simulink library "csc_rsp_radar_sensor_prep_lib"  (R2015b)
settings: Solver=ode45  SolverMode=SingleTasking  StartTime=0.0  StopTime=10.0  RelTol=1e-3
values from neighbouring files (symbols this model uses):
  rsp_ldr1_lander_dcm = rot_angles_to_dcm( [rsp_ldr1_lander_rotz rsp_ldr1_lander_roty rsp_ldr1_lander_rotx] )    [csc_rsp_radar_sensor_prep.m]
  snp_rdr_index = [ 1 2 ]    [csc_snp_sensor_prep_init.m]
  snp_rdr_zero_index = [ 0 0 ]    [csc_snp_sensor_prep_init.m]
undefined symbols (not defined in the file or in its folder): accel, central_body_flattening, central_body_radius, central_body_rotation_rate, ini_topocentric_latitude, kfl_target_site_planet_fixed, kfl_topo_z_to_alt, kfl_use_range_meas, q, x
libraries: util_common_lib x15, simulink x12, util_frame_rotation_lib x7, simulink_extras x6, util_quat_lib x5, util_fsw_frame_rotation_lib x5, util_geodesy_lib x4, util_info_lib x3, csu_und_unduplicate_lib x3, csc_rsp_radar_sensor_prep_lib x2
settings Model: ExtModeAutoUpdateStatusClock=off  Creator=Administrator  LastModifiedBy=Mark Agbayani
settings DataIOCC: SaveFormat=Array  SignalLoggingSaveFormat=ModelDataLogs
settings OptimizationCC: BlockReduction=off  BooleanDataType=off  ExpressionDepthLimit=2147483647
settings DebuggingCC: SaveWithParameterizedLinksMsg=none  UnderspecifiedInitializationDetection=Classic  MergeDetectMultiDrivingBlocksExec=none  SignalResolutionControl=TryResolveAllWithWarning  FcnCallInpInsideContextMsg=EnableAllAsWarning  StateNameClashWarn=warning  StrictBusMsg=Warning
settings HardwareCC: ProdBitPerPointer=32  ProdLargestAtomicFloat=None  ProdIntDivRoundTo=Undefined  ProdEndianess=Unspecified  ProdWordSize=32  ProdHWDeviceType=32-bit Generic  TargetUnknown=on
settings GRTTargetCC: GeneratePreprocessorConditionals=Disable all  CombineOutputUpdateFcns=off  GRTInterface=on
settings ConfigComp: CovModelRefEnable=Off  CovSFcnEnable=off

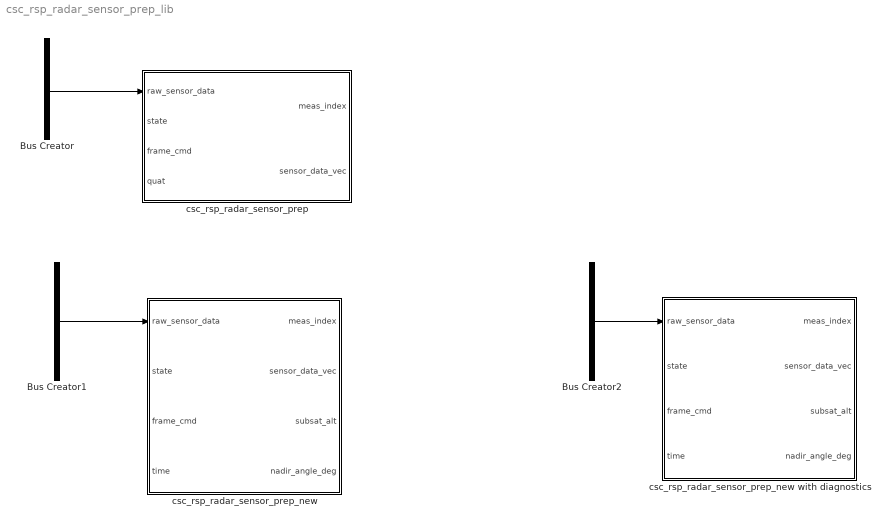
== system csc_rsp_radar_sensor_prep_lib ==
  Bus Creator : BusCreator  Inputs=4
  Bus Creator1 : BusCreator  Inputs=5
  Bus Creator2 : BusCreator  Inputs=5
  csc_rsp_radar_sensor_prep : Subsystem
  csc_rsp_radar_sensor_prep_new : Subsystem
  csc_rsp_radar_sensor_prep_new with diagnostics : Subsystem
  wires:
  ? -> Bus Creator/2  "accel"
  ? -> Bus Creator/3  "rate"
  ? -> Bus Creator/1  "x"
  ? -> Bus Creator/4  "q"
  Bus Creator/1 -> csc_rsp_radar_sensor_prep/1(raw_sensor_data)
  ? -> Bus Creator1/2  "accel"
  ? -> Bus Creator1/3  "rate"
  ? -> Bus Creator1/1  "x"
  ? -> Bus Creator1/4  "q"
  Bus Creator1/1 -> csc_rsp_radar_sensor_prep_new/1(raw_sensor_data)
  ? -> Bus Creator1/5  "altitude"
  ? -> Bus Creator2/2  "accel"
  ? -> Bus Creator2/3  "rate"
  ? -> Bus Creator2/1  "x"
  ? -> Bus Creator2/4  "q"
  Bus Creator2/1 -> csc_rsp_radar_sensor_prep_new with diagnostics/1(raw_sensor_data)
  ? -> Bus Creator2/5  "altitude"

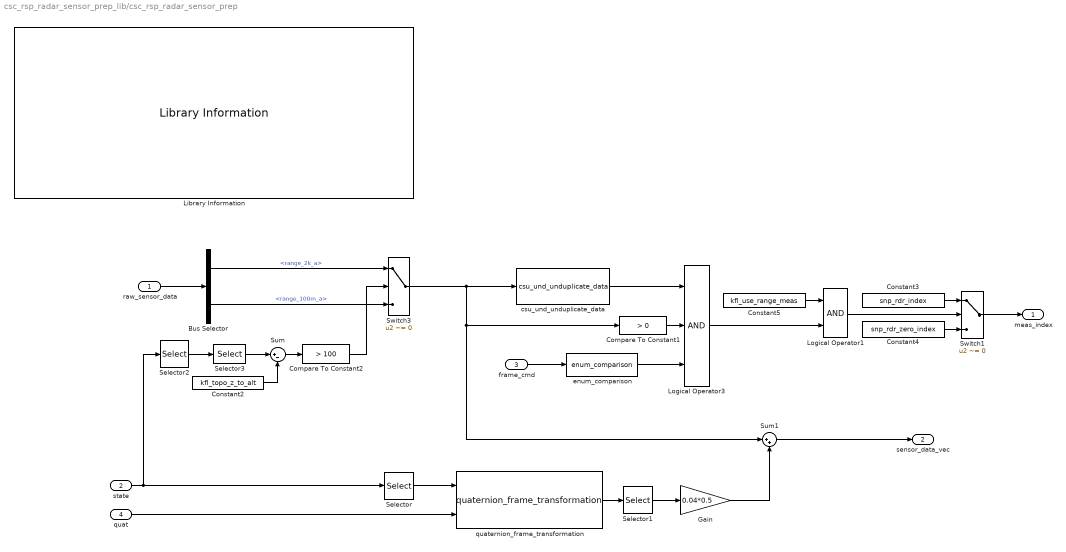
== system csc_rsp_radar_sensor_prep_lib/csc_rsp_radar_sensor_prep ==
  raw_sensor_data : Inport
  state : Inport  Port=2
  frame_cmd : Inport  Port=3
  quat : Inport  Port=4
  Bus Selector : BusSelector  OutputSignals=range_2k_a,range_100m_a
  Compare To Constant1 : simulink/Logic and Bit Operations/Compare To Constant  relop=>  const=0  OutDataTypeStr=uint8
  Compare To Constant2 : simulink/Logic and Bit Operations/Compare To Constant  relop=>  const=100  OutDataTypeStr=uint8
  Constant2 : Constant  Value=kfl_topo_z_to_alt
  Constant3 : Constant  Value=snp_rdr_index
  Constant4 : Constant  Value=snp_rdr_zero_index
  Constant5 : Constant  Value=kfl_use_range_meas
  Gain : Gain  Gain=0.04*0.5
  Library Information : util_info_lib/Library Information  owner='NONE'
  Logical Operator1 : Logic  AllPortsSameDT=off  OutDataTypeStr=boolean
  Logical Operator3 : Logic  Inputs=3  AllPortsSameDT=off  OutDataTypeStr=boolean
  Selector : Selector  InputPortWidth=kfl_n_state  IndexOptions=Index vector (dialog)  Indices=kfl_vel_index  OutputSizes=1
  Selector1 : Selector  InputPortWidth=3  IndexOptions=Index vector (dialog)  Indices=3  OutputSizes=1
  Selector2 : Selector  InputPortWidth=kfl_n_state  IndexOptions=Index vector (dialog)  Indices=kfl_pos_index  OutputSizes=1
  Selector3 : Selector  InputPortWidth=3  IndexOptions=Index vector (dialog)  Indices=[3]  OutputSizes=1
  Sum : Sum  Inputs=|+-
  Sum1 : Sum  Inputs=|++
  Switch1 : Switch  Criteria=u2 ~= 0
  Switch3 : Switch  Criteria=u2 ~= 0
  csu_und_unduplicate_data : csu_und_unduplicate_lib/csu_und_unduplicate_data  initial_compare=0
  enum_comparison : util_common_lib/enum_comparison  comparison_type===
  quaternion_frame_transformation : util_quat_lib/quaternion_frame_transformation  SystemSampleTime=-1
  meas_index : Outport
  sensor_data_vec : Outport  Port=2
  wires:
  csu_und_unduplicate_data/1 -> Logical Operator3/1
  Constant5/1 -> Logical Operator1/1
  Logical Operator1/1 -> Switch1/2
  Logical Operator3/1 -> Logical Operator1/2
  Constant4/1 -> Switch1/3
  Constant3/1 -> Switch1/1
  Switch3/1 -> csu_und_unduplicate_data/1, Compare To Constant1/1, Sum1/1
  Bus Selector/2 -> Switch3/3  "<range_100m_a>"
  Bus Selector/1 -> Switch3/1  "<range_2k_a>"
  Compare To Constant2/1 -> Switch3/2
  Sum/1 -> Compare To Constant2/1
  Selector2/1 -> Selector3/1
  Constant2/1 -> Sum/2
  Selector3/1 -> Sum/1
  Sum1/1 -> sensor_data_vec/1
  Gain/1 -> Sum1/2
  Selector1/1 -> Gain/1
  quaternion_frame_transformation/1 -> Selector1/1
  quat/1 -> quaternion_frame_transformation/2
  Selector/1 -> quaternion_frame_transformation/1
  state/1 -> Selector/1, Selector2/1
  frame_cmd/1 -> enum_comparison/1
  Compare To Constant1/1 -> Logical Operator3/2
  raw_sensor_data/1 -> Bus Selector/1
  Switch1/1 -> meas_index/1
  enum_comparison/1 -> Logical Operator3/3

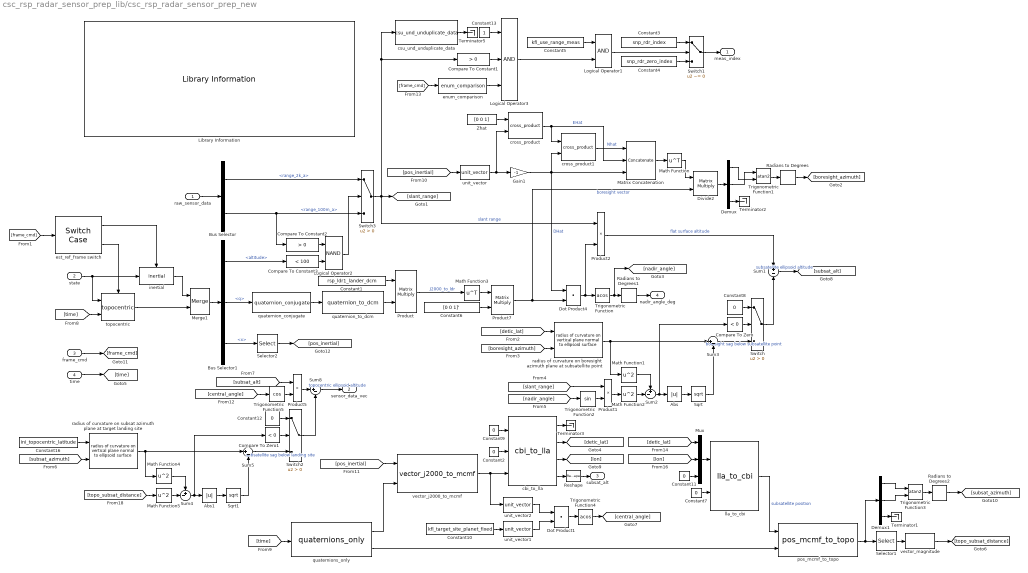
== system csc_rsp_radar_sensor_prep_lib/csc_rsp_radar_sensor_prep_new ==
  raw_sensor_data : Inport
  state : Inport  Port=2
  frame_cmd : Inport  Port=3
  time : Inport  Port=4
  Abs : Abs
  Abs1 : Abs
  Bus Selector : BusSelector  OutputSignals=range_2k_a,range_100m_a
  Bus Selector1 : BusSelector  OutputSignals=altitude,q,x
  Compare To Constant1 : simulink/Logic and Bit Operations/Compare To Constant  relop=>  const=0  OutDataTypeStr=uint8
  Compare To Constant2 : simulink/Logic and Bit Operations/Compare To Constant  relop=>  const=0  OutDataTypeStr=uint8
  Compare To Constant3 : simulink/Logic and Bit Operations/Compare To Constant  relop=<  const=100  OutDataTypeStr=uint8
  Compare To Zero : simulink/Logic and Bit Operations/Compare To Zero  relop=<  OutDataTypeStr=boolean
  Compare To Zero1 : simulink/Logic and Bit Operations/Compare To Zero  relop=<  OutDataTypeStr=boolean
  Constant1 : Constant  Value=rsp_ldr1_lander_dcm
  Constant10 : Constant  Value=kfl_target_site_planet_fixed
  Constant{2,7..9,11..12} (6 alike) : Constant  Value=0
  Constant13 : Constant  OutDataTypeStr=boolean
  Constant16 : Constant  Value=ini_topocentric_latitude
  Constant3 : Constant  Value=snp_rdr_index
  Constant4 : Constant  Value=snp_rdr_zero_index
  Constant5 : Constant  Value=kfl_use_range_meas
  Constant6 : Constant  Value=[0 0 1]'  VectorParams1D=off
  Demux : Demux  Outputs=3
  Demux1 : Demux  Outputs=3
  Divide2 : Product  Inputs=**  Multiplication=Matrix(*)
  Dot Product1 : DotProduct  InputSameDT=on  OutDataTypeStr=Inherit: Inherit via internal rule
  Dot Product4 : DotProduct  InputSameDT=on  OutDataTypeStr=Inherit: Inherit via internal rule
  Gain1 : Gain  Gain=-1
  Library Information : util_info_lib/Library Information  owner='NONE'
  Logical Operator1 : Logic  AllPortsSameDT=off  OutDataTypeStr=boolean
  Logical Operator2 : Logic  Operator=NAND  AllPortsSameDT=off  OutDataTypeStr=boolean
  Logical Operator3 : Logic  Inputs=3  AllPortsSameDT=off  OutDataTypeStr=boolean
  Math Function : Math  Operator=transpose  SaturateOnIntegerOverflow=on
  Math Function{1..2,4..5} (4 alike) : Math  Operator=square  SaturateOnIntegerOverflow=on
  Math Function3 : Math  Operator=transpose  SaturateOnIntegerOverflow=on
  Matrix Concatenation : Concatenate  NumInputs=3  Mode=Multidimensional array  ConcatenateDimension=2
  Merge1 : Merge  InitialOutput=0
  Mux : Mux  Inputs=3
  Product : Product  Multiplication=Matrix(*)  RndMeth=Zero
  Product1 : Product  Inputs=**  RndMeth=Zero
  Product2 : Product  Inputs=**  RndMeth=Zero
  Product5 : Product  Inputs=**  RndMeth=Zero
  Product7 : Product  Multiplication=Matrix(*)  RndMeth=Zero
  Radians to Degrees : simulink_extras/Transformations/Radians to Degrees
  Radians to Degrees1 : simulink_extras/Transformations/Radians to Degrees
  Radians to Degrees2 : simulink_extras/Transformations/Radians to Degrees
  Reshape : Reshape
  Selector1 : Selector  InputPortWidth=3  IndexOptions=Index vector (dialog)  Indices=[1 2]  OutputSizes=1
  Selector2 : Selector  InputPortWidth=kfl_n_state  IndexOptions=Index vector (dialog)  Indices=kfl_pos_index  OutputSizes=1
  Sqrt : Sqrt  SaturateOnIntegerOverflow=on
  Sqrt1 : Sqrt  SaturateOnIntegerOverflow=on
  Sum1 : Sum  Inputs=+|-
  Sum2 : Sum  Inputs=+-|  AccumDataTypeStr=double
  Sum3 : Sum  Inputs=|+-
  Sum4 : Sum  Inputs=+-|  AccumDataTypeStr=double
  Sum5 : Sum  Inputs=|+-
  Sum8 : Sum  Inputs=|+-
  Switch : Switch  Criteria=u2 > Threshold
  Switch1 : Switch  Criteria=u2 ~= 0
  Switch2 : Switch  Criteria=u2 > Threshold
  Switch3 : Switch  Criteria=u2 > Threshold
  Terminator{1..3,5} (4 alike) : Terminator
  Trigonometric Function : Trigonometry  Operator=acos
  Trigonometric Function1 : Trigonometry  Operator=atan2
  Trigonometric Function2 : Trigonometry
  Trigonometric Function3 : Trigonometry  Operator=atan2
  Trigonometric Function4 : Trigonometry  Operator=acos
  Trigonometric Function5 : Trigonometry  Operator=cos
  Zhat : Constant  Value=[0 0 1]
  cbi_to_lla : util_frame_rotation_lib/cbi_to_lla  a=central_body_radius  b=central_body_radius*(1-central_body_flattening)  omega=central_body_rotation_rate(3)
  cross_product : util_common_lib/cross_product  SystemSampleTime=-1
  cross_product1 : util_common_lib/cross_product  SystemSampleTime=-1
  csu_und_unduplicate_data : csu_und_unduplicate_lib/csu_und_unduplicate_data  initial_compare=0
  enum_comparison : util_common_lib/enum_comparison  comparison_type===
  est_ref_frame switch : SwitchCase  CaseConditions={uint8(enum_reference_frame.inertial),uint8(enum_reference_frame.topocentric)}  ShowDefaultCase=off
  inertial : csc_rsp_radar_sensor_prep_lib/csc_rsp_radar_sensor_prep_new with diagnostics/inertial
  lla_to_cbi : util_frame_rotation_lib/lla_to_cbi  a=central_body_radius  b=central_body_radius*(1-central_body_flattening)
  pos_mcmf_to_topo : util_fsw_frame_rotation_lib/pos_mcmf_to_topo  SystemSampleTime=-1
  quaternion_conjugate : util_quat_lib/quaternion_conjugate  SystemSampleTime=-1
  quaternion_to_dcm : util_quat_lib/quaternion_to_dcm  SystemSampleTime=-1
  quaternions_only : util_frame_rotation_lib/quaternions_only  SystemSampleTime=-1
  radius of curvature on boresight azimuth plane at subsatellite point : util_geodesy_lib/radius of curvature on vertical plane normal to ellipsoid surface  a=central_body_radius  b=central_body_radius*(1-central_body_flattening)
  radius of curvature on subsat azimuth plane at target landing site : util_geodesy_lib/radius of curvature on vertical plane normal to ellipsoid surface  a=central_body_radius  b=central_body_radius*(1-central_body_flattening)
  topocentric : csc_rsp_radar_sensor_prep_lib/csc_rsp_radar_sensor_prep_new with diagnostics/topocentric
  unit_vector : util_common_lib/unit_vector  SystemSampleTime=-1
  unit_vector1 : util_common_lib/unit_vector  SystemSampleTime=-1
  unit_vector2 : util_common_lib/unit_vector  SystemSampleTime=-1
  vector_j2000_to_mcmf : util_fsw_frame_rotation_lib/vector_j2000_to_mcmf  SystemSampleTime=-1
  vector_magnitude : util_common_lib/vector_magnitude  SystemSampleTime=-1
  meas_index : Outport
  sensor_data_vec : Outport  Port=2
  subsat_alt : Outport  Port=3
  nadir_angle_deg : Outport  Port=4
  wires:
  Reshape/1 -> subsat_alt/1
  Switch3/1 -> [slant_range], csu_und_unduplicate_data/1, Compare To Constant1/1, Product2/1  "slant range"
  unit_vector2/1 -> Dot Product1/1
  [pos_inertial] -> unit_vector/1
  Selector2/1 -> [pos_inertial]
  [pos_inertial] -> vector_j2000_to_mcmf/1
  unit_vector1/1 -> Dot Product1/2
  Constant11/1 -> Mux/3
  [detic_lat] -> Mux/1
  [lon] -> Mux/2
  cbi_to_lla/2 -> [detic_lat]
  cbi_to_lla/3 -> [lon]
  cbi_to_lla/1 -> Terminator3/1
  Constant9/1 -> cbi_to_lla/1
  Constant2/1 -> cbi_to_lla/2
  vector_j2000_to_mcmf/1 -> cbi_to_lla/3, unit_vector2/1
  [subsat_azimuth] -> radius of curvature on subsat azimuth plane at target landing site/2
  Demux1/2 -> Trigonometric Function3/2
  Demux1/1 -> Trigonometric Function3/1
  Radians to Degrees2/1 -> [subsat_azimuth]
  pos_mcmf_to_topo/1 -> Selector1/1, Demux1/1
  Demux1/3 -> Terminator1/1
  Trigonometric Function3/1 -> Radians to Degrees2/1
  Constant16/1 -> radius of curvature on subsat azimuth plane at target landing site/1
  Constant7/1 -> lla_to_cbi/2
  cbi_to_lla/4 -> Reshape/1
  Mux/1 -> lla_to_cbi/1
  vector_magnitude/1 -> [topo_subsat_distance]
  lla_to_cbi/1 -> pos_mcmf_to_topo/1  "subsatellite position"
  Compare To Constant3/1 -> Logical Operator2/2
  Compare To Constant2/1 -> Logical Operator2/1
  Constant13/1 -> Logical Operator3/1
  csu_und_unduplicate_data/1 -> Terminator5/1
  quaternions_only/2 -> pos_mcmf_to_topo/2
  quaternions_only/1 -> vector_j2000_to_mcmf/2
  Selector1/1 -> vector_magnitude/1
  Trigonometric Function4/1 -> [central_angle]
  Switch2/1 -> Sum8/2
  Product5/1 -> Sum8/1
  [central_angle] -> Trigonometric Function5/1
  [subsat_alt] -> Product5/1
  Trigonometric Function5/1 -> Product5/2
  Constant10/1 -> unit_vector1/1
  Dot Product1/1 -> Trigonometric Function4/1
  [topo_subsat_distance] -> Math Function5/1
  Sum4/1 -> Abs1/1, Compare To Zero1/1
  Abs1/1 -> Sqrt1/1
  Constant12/1 -> Switch2/1
  Compare To Zero1/1 -> Switch2/2
  Sum5/1 -> Switch2/3  "subsatellite sag below landing site"
  Sqrt1/1 -> Sum5/2
  Math Function5/1 -> Sum4/2
  Math Function4/1 -> Sum4/1
  radius of curvature on subsat azimuth plane at target landing site/1 -> Sum5/1, Math Function4/1
  Switch1/1 -> meas_index/1
  time/1 -> [time]
  Sum8/1 -> sensor_data_vec/1  "topocentric ellipsoid altitude"
  [time] -> quaternions_only/1
  unit_vector/1 -> cross_product/2, Gain1/1
  Switch/1 -> Sum1/2
  Sum2/1 -> Compare To Zero/1, Abs/1
  Abs/1 -> Sqrt/1
  Constant8/1 -> Switch/1
  Compare To Zero/1 -> Switch/2
  Sum3/1 -> Switch/3  "boresight sag below subsatellite point"
  Sum1/1 -> [subsat_alt]  "subsatellite ellipsoid altitude"
  [slant_range] -> Product1/1
  Product1/1 -> Math Function2/1
  Trigonometric Function2/1 -> Product1/2
  [nadir_angle] -> Trigonometric Function2/1
  Sqrt/1 -> Sum3/2
  Math Function2/1 -> Sum2/2
  Math Function1/1 -> Sum2/1
  radius of curvature on boresight azimuth plane at subsatellite point/1 -> Math Function1/1, Sum3/1
  Radians to Degrees/1 -> [boresight_azimuth]
  Product7/1 -> Dot Product4/2, Divide2/2  "boresight vector"
  [boresight_azimuth] -> radius of curvature on boresight azimuth plane at subsatellite point/2
  [detic_lat] -> radius of curvature on boresight azimuth plane at subsatellite point/1
  Gain1/1 -> Matrix Concatenation/3, Dot Product4/1, cross_product1/2  "DHat"
  cross_product/1 -> Matrix Concatenation/2, cross_product1/1  "EHat"
  cross_product1/1 -> Matrix Concatenation/1  "Nhat"
  Matrix Concatenation/1 -> Math Function/1
  Zhat/1 -> cross_product/1
  Math Function/1 -> Divide2/1
  Divide2/1 -> Demux/1
  Demux/3 -> Terminator2/1
  Trigonometric Function1/1 -> Radians to Degrees/1
  Demux/1 -> Trigonometric Function1/2
  Demux/2 -> Trigonometric Function1/1
  Product2/1 -> Sum1/1  "flat surface altitude"
  [frame_cmd] -> enum_comparison/1
  frame_cmd/1 -> [frame_cmd]
  Merge1/1 -> Bus Selector1/1
  [time] -> topocentric/2
  est_ref_frame switch/2 -> topocentric/Action
  topocentric/1 -> Merge1/2
  inertial/1 -> Merge1/1
  state/1 -> inertial/1, topocentric/1
  est_ref_frame switch/1 -> inertial/Action
  [frame_cmd] -> est_ref_frame switch/1
  Radians to Degrees1/1 -> nadir_angle_deg/1
  Trigonometric Function/1 -> Radians to Degrees1/1, [nadir_angle]
  Dot Product4/1 -> Trigonometric Function/1, Product2/2
  quaternion_conjugate/1 -> quaternion_to_dcm/1
  Constant6/1 -> Product7/2
  Constant1/1 -> Product/1
  quaternion_to_dcm/1 -> Product/2
  Math Function3/1 -> Product7/1
  Product/1 -> Math Function3/1  "J2000_to_ldr"
  Constant5/1 -> Logical Operator1/1
  Logical Operator1/1 -> Switch1/2
  Logical Operator3/1 -> Logical Operator1/2
  Constant4/1 -> Switch1/3
  Constant3/1 -> Switch1/1
  Bus Selector/2 -> Switch3/3, Compare To Constant2/1  "<range_100m_a>"
  Bus Selector/1 -> Switch3/1  "<range_2k_a>"
  Logical Operator2/1 -> Switch3/2
  Bus Selector1/1 -> Compare To Constant3/1  "<altitude>"
  Bus Selector1/2 -> quaternion_conjugate/1  "<q>"
  Bus Selector1/3 -> Selector2/1  "<x>"
  Compare To Constant1/1 -> Logical Operator3/2
  raw_sensor_data/1 -> Bus Selector/1
  enum_comparison/1 -> Logical Operator3/3

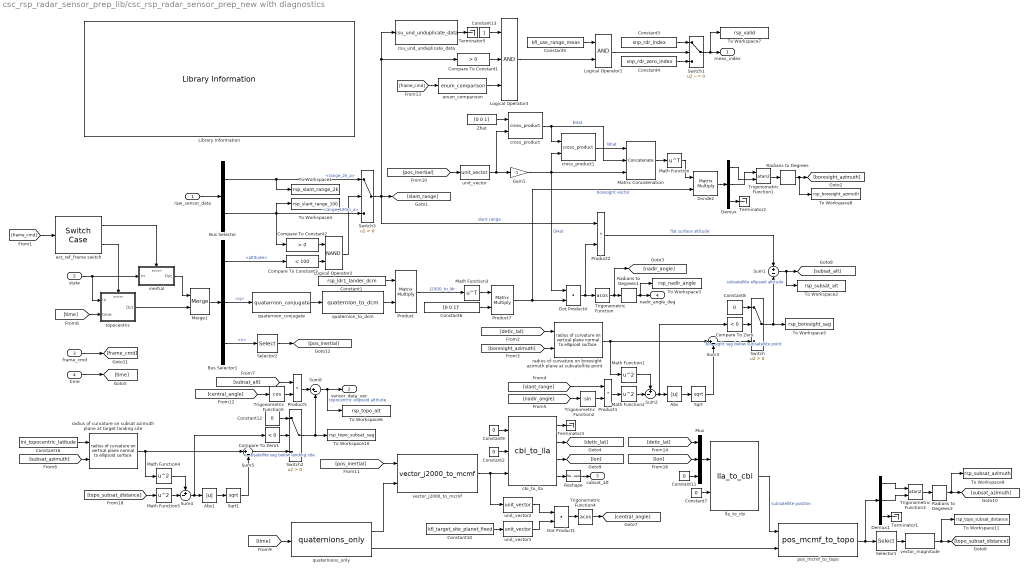
== system csc_rsp_radar_sensor_prep_lib/csc_rsp_radar_sensor_prep_new with diagnostics ==
  raw_sensor_data : Inport
  state : Inport  Port=2
  frame_cmd : Inport  Port=3
  time : Inport  Port=4
  Abs : Abs
  Abs1 : Abs
  Bus Selector : BusSelector  OutputSignals=range_2k_a,range_100m_a
  Bus Selector1 : BusSelector  OutputSignals=altitude,q,x
  Compare To Constant1 : simulink/Logic and Bit Operations/Compare To Constant  relop=>  const=0  OutDataTypeStr=uint8
  Compare To Constant2 : simulink/Logic and Bit Operations/Compare To Constant  relop=>  const=0  OutDataTypeStr=uint8
  Compare To Constant3 : simulink/Logic and Bit Operations/Compare To Constant  relop=<  const=100  OutDataTypeStr=uint8
  Compare To Zero : simulink/Logic and Bit Operations/Compare To Zero  relop=<  OutDataTypeStr=boolean
  Compare To Zero1 : simulink/Logic and Bit Operations/Compare To Zero  relop=<  OutDataTypeStr=boolean
  Constant1 : Constant  Value=rsp_ldr1_lander_dcm
  Constant10 : Constant  Value=kfl_target_site_planet_fixed
  Constant{2,7..9,11..12} (6 alike) : Constant  Value=0
  Constant13 : Constant  OutDataTypeStr=boolean
  Constant16 : Constant  Value=ini_topocentric_latitude
  Constant3 : Constant  Value=snp_rdr_index
  Constant4 : Constant  Value=snp_rdr_zero_index
  Constant5 : Constant  Value=kfl_use_range_meas
  Constant6 : Constant  Value=[0 0 1]'  VectorParams1D=off
  Demux : Demux  Outputs=3
  Demux1 : Demux  Outputs=3
  Divide2 : Product  Inputs=**  Multiplication=Matrix(*)
  Dot Product1 : DotProduct  InputSameDT=on  OutDataTypeStr=Inherit: Inherit via internal rule
  Dot Product4 : DotProduct  InputSameDT=on  OutDataTypeStr=Inherit: Inherit via internal rule
  Gain1 : Gain  Gain=-1
  Library Information : util_info_lib/Library Information  owner='NONE'
  Logical Operator1 : Logic  AllPortsSameDT=off  OutDataTypeStr=boolean
  Logical Operator2 : Logic  Operator=NAND  AllPortsSameDT=off  OutDataTypeStr=boolean
  Logical Operator3 : Logic  Inputs=3  AllPortsSameDT=off  OutDataTypeStr=boolean
  Math Function : Math  Operator=transpose  SaturateOnIntegerOverflow=on
  Math Function{1..2,4..5} (4 alike) : Math  Operator=square  SaturateOnIntegerOverflow=on
  Math Function3 : Math  Operator=transpose  SaturateOnIntegerOverflow=on
  Matrix Concatenation : Concatenate  NumInputs=3  Mode=Multidimensional array  ConcatenateDimension=2
  Merge1 : Merge  InitialOutput=0
  Mux : Mux  Inputs=3
  Product : Product  Multiplication=Matrix(*)  RndMeth=Zero
  Product1 : Product  Inputs=**  RndMeth=Zero
  Product2 : Product  Inputs=**  RndMeth=Zero
  Product5 : Product  Inputs=**  RndMeth=Zero
  Product7 : Product  Multiplication=Matrix(*)  RndMeth=Zero
  Radians to Degrees : simulink_extras/Transformations/Radians to Degrees
  Radians to Degrees1 : simulink_extras/Transformations/Radians to Degrees
  Radians to Degrees2 : simulink_extras/Transformations/Radians to Degrees
  Reshape : Reshape
  Selector1 : Selector  InputPortWidth=3  IndexOptions=Index vector (dialog)  Indices=[1 2]  OutputSizes=1
  Selector2 : Selector  InputPortWidth=kfl_n_state  IndexOptions=Index vector (dialog)  Indices=kfl_pos_index  OutputSizes=1
  Sqrt : Sqrt  SaturateOnIntegerOverflow=on
  Sqrt1 : Sqrt  SaturateOnIntegerOverflow=on
  Sum1 : Sum  Inputs=+|-
  Sum2 : Sum  Inputs=+-|  AccumDataTypeStr=double
  Sum3 : Sum  Inputs=|+-
  Sum4 : Sum  Inputs=+-|  AccumDataTypeStr=double
  Sum5 : Sum  Inputs=|+-
  Sum8 : Sum  Inputs=|+-
  Switch : Switch  Criteria=u2 > Threshold
  Switch1 : Switch  Criteria=u2 ~= 0
  Switch2 : Switch  Criteria=u2 > Threshold
  Switch3 : Switch  Criteria=u2 > Threshold
  Terminator{1..3,5} (4 alike) : Terminator
  To Workspace1 : ToWorkspace  VariableName=rsp_slant_range_2k  SaveFormat=Structure With Time  SampleTime=-1
  To Workspace10 : ToWorkspace  VariableName=rsp_topo_subsat_sag  SaveFormat=Structure With Time  SampleTime=-1
  To Workspace11 : ToWorkspace  VariableName=rsp_topo_subsat_distance  SaveFormat=Structure With Time  SampleTime=-1
  To Workspace2 : ToWorkspace  VariableName=rsp_subsat_alt  SaveFormat=Structure With Time  SampleTime=-1
  To Workspace3 : ToWorkspace  VariableName=rsp_nadir_angle  SaveFormat=Structure With Time  SampleTime=-1
  To Workspace4 : ToWorkspace  VariableName=rsp_slant_range_100  SaveFormat=Structure With Time  SampleTime=-1
  To Workspace5 : ToWorkspace  VariableName=rsp_boresight_sag  SaveFormat=Structure With Time  SampleTime=-1
  To Workspace6 : ToWorkspace  VariableName=rsp_topo_alt  SaveFormat=Structure With Time  SampleTime=-1
  To Workspace7 : ToWorkspace  VariableName=rsp_valid  SaveFormat=Structure With Time  SampleTime=-1
  To Workspace8 : ToWorkspace  VariableName=rsp_boresight_azimuth  SaveFormat=Structure With Time  SampleTime=-1
  To Workspace9 : ToWorkspace  VariableName=rsp_subsat_azimuth  SaveFormat=Structure With Time  SampleTime=-1
  Trigonometric Function : Trigonometry  Operator=acos
  Trigonometric Function1 : Trigonometry  Operator=atan2
  Trigonometric Function2 : Trigonometry
  Trigonometric Function3 : Trigonometry  Operator=atan2
  Trigonometric Function4 : Trigonometry  Operator=acos
  Trigonometric Function5 : Trigonometry  Operator=cos
  Zhat : Constant  Value=[0 0 1]
  cbi_to_lla : util_frame_rotation_lib/cbi_to_lla  a=central_body_radius  b=central_body_radius*(1-central_body_flattening)  omega=central_body_rotation_rate(3)
  cross_product : util_common_lib/cross_product  SystemSampleTime=-1
  cross_product1 : util_common_lib/cross_product  SystemSampleTime=-1
  csu_und_unduplicate_data : csu_und_unduplicate_lib/csu_und_unduplicate_data  initial_compare=0
  enum_comparison : util_common_lib/enum_comparison  comparison_type===
  est_ref_frame switch : SwitchCase  CaseConditions={uint8(enum_reference_frame.inertial),uint8(enum_reference_frame.topocentric)}  ShowDefaultCase=off
  inertial : Subsystem  TreatAsAtomicUnit=on
  lla_to_cbi : util_frame_rotation_lib/lla_to_cbi  a=central_body_radius  b=central_body_radius*(1-central_body_flattening)
  pos_mcmf_to_topo : util_fsw_frame_rotation_lib/pos_mcmf_to_topo  SystemSampleTime=-1
  quaternion_conjugate : util_quat_lib/quaternion_conjugate  SystemSampleTime=-1
  quaternion_to_dcm : util_quat_lib/quaternion_to_dcm  SystemSampleTime=-1
  quaternions_only : util_frame_rotation_lib/quaternions_only  SystemSampleTime=-1
  radius of curvature on boresight azimuth plane at subsatellite point : util_geodesy_lib/radius of curvature on vertical plane normal to ellipsoid surface  a=central_body_radius  b=central_body_radius*(1-central_body_flattening)
  radius of curvature on subsat azimuth plane at target landing site : util_geodesy_lib/radius of curvature on vertical plane normal to ellipsoid surface  a=central_body_radius  b=central_body_radius*(1-central_body_flattening)
  topocentric : Subsystem  TreatAsAtomicUnit=on
  unit_vector : util_common_lib/unit_vector  SystemSampleTime=-1
  unit_vector1 : util_common_lib/unit_vector  SystemSampleTime=-1
  unit_vector2 : util_common_lib/unit_vector  SystemSampleTime=-1
  vector_j2000_to_mcmf : util_fsw_frame_rotation_lib/vector_j2000_to_mcmf  SystemSampleTime=-1
  vector_magnitude : util_common_lib/vector_magnitude  SystemSampleTime=-1
  meas_index : Outport
  sensor_data_vec : Outport  Port=2
  subsat_alt : Outport  Port=3
  nadir_angle_deg : Outport  Port=4
  wires:
  Reshape/1 -> subsat_alt/1
  Switch3/1 -> [slant_range], csu_und_unduplicate_data/1, Compare To Constant1/1, Product2/1  "slant range"
  unit_vector2/1 -> Dot Product1/1
  [pos_inertial] -> unit_vector/1
  Selector2/1 -> [pos_inertial]
  [pos_inertial] -> vector_j2000_to_mcmf/1
  unit_vector1/1 -> Dot Product1/2
  Constant11/1 -> Mux/3
  [detic_lat] -> Mux/1
  [lon] -> Mux/2
  cbi_to_lla/2 -> [detic_lat]
  cbi_to_lla/3 -> [lon]
  cbi_to_lla/1 -> Terminator3/1
  Constant9/1 -> cbi_to_lla/1
  Constant2/1 -> cbi_to_lla/2
  vector_j2000_to_mcmf/1 -> cbi_to_lla/3, unit_vector2/1
  [subsat_azimuth] -> radius of curvature on subsat azimuth plane at target landing site/2
  Demux1/2 -> Trigonometric Function3/2
  Demux1/1 -> Trigonometric Function3/1
  Radians to Degrees2/1 -> [subsat_azimuth], To Workspace9/1
  pos_mcmf_to_topo/1 -> Selector1/1, Demux1/1
  Demux1/3 -> Terminator1/1
  Trigonometric Function3/1 -> Radians to Degrees2/1
  Constant16/1 -> radius of curvature on subsat azimuth plane at target landing site/1
  Constant7/1 -> lla_to_cbi/2
  cbi_to_lla/4 -> Reshape/1
  Mux/1 -> lla_to_cbi/1
  vector_magnitude/1 -> To Workspace11/1, [topo_subsat_distance]
  lla_to_cbi/1 -> pos_mcmf_to_topo/1  "subsatellite position"
  Compare To Constant3/1 -> Logical Operator2/2
  Compare To Constant2/1 -> Logical Operator2/1
  Constant13/1 -> Logical Operator3/1
  csu_und_unduplicate_data/1 -> Terminator5/1
  quaternions_only/2 -> pos_mcmf_to_topo/2
  quaternions_only/1 -> vector_j2000_to_mcmf/2
  Selector1/1 -> vector_magnitude/1
  Trigonometric Function4/1 -> [central_angle]
  Switch2/1 -> Sum8/2, To Workspace10/1
  Product5/1 -> Sum8/1
  [central_angle] -> Trigonometric Function5/1
  [subsat_alt] -> Product5/1
  Trigonometric Function5/1 -> Product5/2
  Constant10/1 -> unit_vector1/1
  Dot Product1/1 -> Trigonometric Function4/1
  [topo_subsat_distance] -> Math Function5/1
  Sum4/1 -> Abs1/1, Compare To Zero1/1
  Abs1/1 -> Sqrt1/1
  Constant12/1 -> Switch2/1
  Compare To Zero1/1 -> Switch2/2
  Sum5/1 -> Switch2/3  "subsatellite sag below landing site"
  Sqrt1/1 -> Sum5/2
  Math Function5/1 -> Sum4/2
  Math Function4/1 -> Sum4/1
  radius of curvature on subsat azimuth plane at target landing site/1 -> Sum5/1, Math Function4/1
  Switch1/1 -> meas_index/1, To Workspace7/1
  time/1 -> [time]
  Sum8/1 -> sensor_data_vec/1, To Workspace6/1  "topocentric ellipsoid altitude"
  [time] -> quaternions_only/1
  unit_vector/1 -> cross_product/2, Gain1/1
  Switch/1 -> Sum1/2, To Workspace5/1
  Sum2/1 -> Compare To Zero/1, Abs/1
  Abs/1 -> Sqrt/1
  Constant8/1 -> Switch/1
  Compare To Zero/1 -> Switch/2
  Sum3/1 -> Switch/3  "boresight sag below subsatellite point"
  Sum1/1 -> [subsat_alt], To Workspace2/1  "subsatellite ellipsoid altitude"
  [slant_range] -> Product1/1
  Product1/1 -> Math Function2/1
  Trigonometric Function2/1 -> Product1/2
  [nadir_angle] -> Trigonometric Function2/1
  Sqrt/1 -> Sum3/2
  Math Function2/1 -> Sum2/2
  Math Function1/1 -> Sum2/1
  radius of curvature on boresight azimuth plane at subsatellite point/1 -> Math Function1/1, Sum3/1
  Radians to Degrees/1 -> [boresight_azimuth], To Workspace8/1
  Product7/1 -> Dot Product4/2, Divide2/2  "boresight vector"
  [boresight_azimuth] -> radius of curvature on boresight azimuth plane at subsatellite point/2
  [detic_lat] -> radius of curvature on boresight azimuth plane at subsatellite point/1
  Gain1/1 -> Matrix Concatenation/3, Dot Product4/1, cross_product1/2  "DHat"
  cross_product/1 -> Matrix Concatenation/2, cross_product1/1  "EHat"
  cross_product1/1 -> Matrix Concatenation/1  "Nhat"
  Matrix Concatenation/1 -> Math Function/1
  Zhat/1 -> cross_product/1
  Math Function/1 -> Divide2/1
  Divide2/1 -> Demux/1
  Demux/3 -> Terminator2/1
  Trigonometric Function1/1 -> Radians to Degrees/1
  Demux/1 -> Trigonometric Function1/2
  Demux/2 -> Trigonometric Function1/1
  Product2/1 -> Sum1/1  "flat surface altitude"
  [frame_cmd] -> enum_comparison/1
  frame_cmd/1 -> [frame_cmd]
  Merge1/1 -> Bus Selector1/1
  [time] -> topocentric/2(time)
  est_ref_frame switch/2 -> topocentric/Action
  topocentric/1(Out) -> Merge1/2
  inertial/1(Out) -> Merge1/1
  state/1 -> inertial/1(In), topocentric/1(In)
  est_ref_frame switch/1 -> inertial/Action
  [frame_cmd] -> est_ref_frame switch/1
  Radians to Degrees1/1 -> nadir_angle_deg/1, To Workspace3/1
  Trigonometric Function/1 -> Radians to Degrees1/1, [nadir_angle]
  Dot Product4/1 -> Trigonometric Function/1, Product2/2
  quaternion_conjugate/1 -> quaternion_to_dcm/1
  Constant6/1 -> Product7/2
  Constant1/1 -> Product/1
  quaternion_to_dcm/1 -> Product/2
  Math Function3/1 -> Product7/1
  Product/1 -> Math Function3/1  "J2000_to_ldr"
  Constant5/1 -> Logical Operator1/1
  Logical Operator1/1 -> Switch1/2
  Logical Operator3/1 -> Logical Operator1/2
  Constant4/1 -> Switch1/3
  Constant3/1 -> Switch1/1
  Bus Selector/2 -> Switch3/3, Compare To Constant2/1, To Workspace4/1  "<range_100m_a>"
  Bus Selector/1 -> Switch3/1, To Workspace1/1  "<range_2k_a>"
  Logical Operator2/1 -> Switch3/2
  Bus Selector1/1 -> Compare To Constant3/1  "<altitude>"
  Bus Selector1/2 -> quaternion_conjugate/1  "<q>"
  Bus Selector1/3 -> Selector2/1  "<x>"
  Compare To Constant1/1 -> Logical Operator3/2
  raw_sensor_data/1 -> Bus Selector/1
  enum_comparison/1 -> Logical Operator3/3

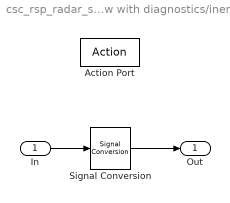
== system csc_rsp_radar_sensor_prep_lib/csc_rsp_radar_sensor_prep_new with diagnostics/inertial ==
  In : Inport
  Action Port : ActionPort
  Signal Conversion : SignalConversion
  Out : Outport
  wires:
  Signal Conversion/1 -> Out/1
  In/1 -> Signal Conversion/1

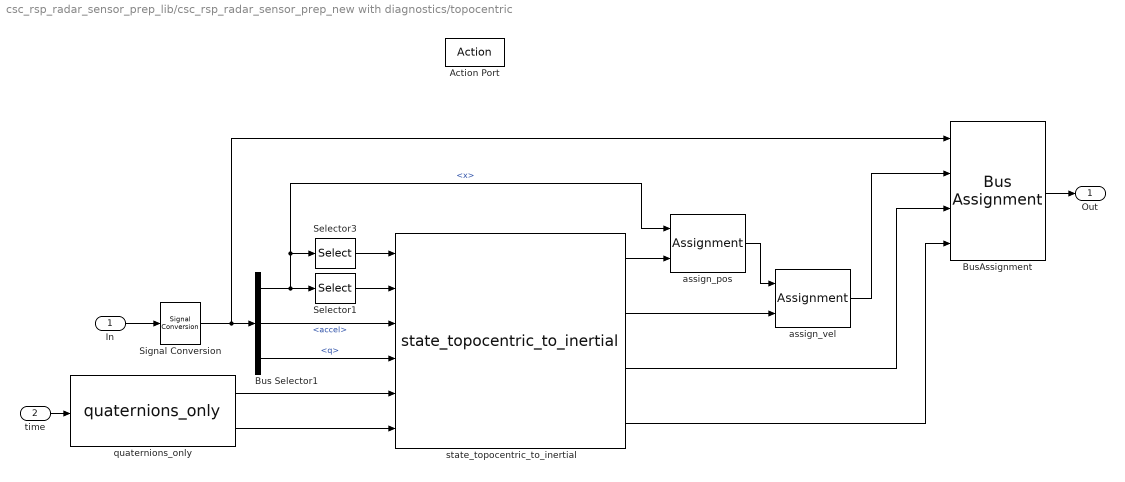
== system csc_rsp_radar_sensor_prep_lib/csc_rsp_radar_sensor_prep_new with diagnostics/topocentric ==
  In : Inport
  time : Inport  Port=2
  Action Port : ActionPort
  Bus Selector1 : BusSelector  OutputSignals=x,accel,q
  BusAssignment : BusAssignment  AssignedSignals=x,accel,q
  Selector1 : Selector  InputPortWidth=kfl_n_state  IndexOptions=Index vector (dialog)  Indices=kfl_vel_index  OutputSizes=1
  Selector3 : Selector  InputPortWidth=kfl_n_state  IndexOptions=Index vector (dialog)  Indices=kfl_pos_index  OutputSizes=1
  Signal Conversion : SignalConversion
  assign_pos : Assignment  IndexOptions=Index vector (dialog)  Indices=kfl_pos_index  OutputSizes=1
  assign_vel : Assignment  IndexOptions=Index vector (dialog)  Indices=kfl_vel_index  OutputSizes=1
  quaternions_only : util_frame_rotation_lib/quaternions_only  SystemSampleTime=-1
  state_topocentric_to_inertial : util_fsw_frame_rotation_lib/state_topocentric_to_inertial  SystemSampleTime=-1
  Out : Outport
  wires:
  Signal Conversion/1 -> Bus Selector1/1, BusAssignment/1
  In/1 -> Signal Conversion/1
  assign_vel/1 -> BusAssignment/2
  state_topocentric_to_inertial/2 -> assign_vel/2
  assign_pos/1 -> assign_vel/1
  state_topocentric_to_inertial/1 -> assign_pos/2
  Bus Selector1/3 -> state_topocentric_to_inertial/4  "<q>"
  Bus Selector1/2 -> state_topocentric_to_inertial/3  "<accel>"
  Selector1/1 -> state_topocentric_to_inertial/2
  Selector3/1 -> state_topocentric_to_inertial/1
  Bus Selector1/1 -> Selector1/1, Selector3/1, assign_pos/1  "<x>"
  quaternions_only/2 -> state_topocentric_to_inertial/6
  quaternions_only/1 -> state_topocentric_to_inertial/5
  time/1 -> quaternions_only/1
  BusAssignment/1 -> Out/1
  state_topocentric_to_inertial/4 -> BusAssignment/4
  state_topocentric_to_inertial/3 -> BusAssignment/3
